simulink model "AIM_v0"  (R2015a)
settings: Solver=ode4  SolverMode=SingleTasking  StartTime=0.0  StopTime=stop_time  FixedStep=1  RelTol=1e-3
undefined symbols (not defined in the file or in its folder): slcm, Target
undefined symbols (not defined in the file): Chaser, Constant
libraries: lib_gravity x6, RotationalDynamics x4, vrlib x3, TranslationalDynamics3DoF x2, Ephemeris_reader x1, Disturbances x1, visualisation x1
settings Model: Creator=bbrito  LastModifiedBy=bbrito
settings DataIOCC: SignalLoggingSaveFormat=ModelDataLogs
settings OptimizationCC: BlockReduction=off  BooleanDataType=off
settings DebuggingCC: SaveWithParameterizedLinksMsg=none  UnderspecifiedInitializationDetection=Classic  MergeDetectMultiDrivingBlocksExec=none  SignalResolutionControl=TryResolveAllWithWarning  MultiTaskDSMMsg=warning  MultiTaskCondExecSysMsg=none
settings HardwareCC: TargetUnknown=on

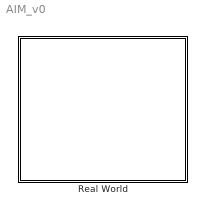
== system AIM_v0 ==
  Real World : Subsystem  TreatAsAtomicUnit=on

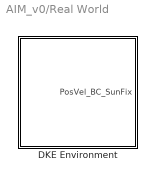
== system AIM_v0/Real World ==
  "DKE Environment " : Subsystem  TreatAsAtomicUnit=on

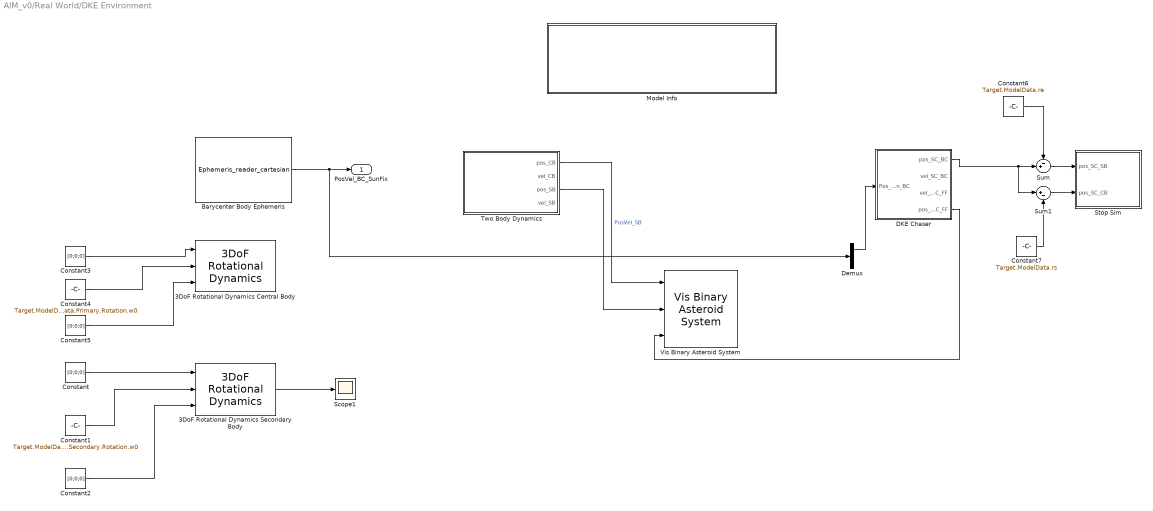
== system AIM_v0/Real World/DKE Environment  ==
  3DoF Rotational Dynamics Central Body : RotationalDynamics/3DoF Rotational Dynamics  I=Target.ModelData.Primary.I
  3DoF Rotational Dynamics Secondary Body : RotationalDynamics/3DoF Rotational Dynamics  I=Target.ModelData.Secondary.I
  Barycenter Body Ephemeris : Ephemeris_reader/Ephemeris_reader_cartesian  traj=Target.ModelData.Primary.Trajectory
  Constant{,2..3,5} (4 alike) : Constant  Value=[0;0;0]
  Constant1 : Constant  Value=Target.ModelData.Secondary.Rotation.w0
  Constant4 : Constant  Value=Target.ModelData.Primary.Rotation.w0
  Constant6 : Constant  Value=Target.ModelData.re
  Constant7 : Constant  Value=Target.ModelData.rs
  DKE Chaser : Subsystem  TreatAsAtomicUnit=on
  Demux : Demux  Outputs=2
  Model Info : Subsystem  LoadFcn=slcm LoadBlock;  InitFcn=slcm('UpdateAllCMBlocksInThisModelInit')  mask(CMBlock){InitialSaveTempField=, InitialBlockCM=, BlockCM=, Frame=on, SaveTempField=, DisplayStringWithTags=|, MaskDisplayString=Copyright ESA, S.A. 2015.\n---------------------------------------------------------------------------\nVersion:0.0          Date:9/11/2015          Author: #BB\nMatlab Ver.: MATLAB 2015a          Project:AIM          Section:TEC-ECN\n---------------------------------------------------------------------------\nAIM target dynamics, HorizontalTextAlignment=Center, LeftAlignmentValue=0.5, SourceBlockDiagram=AIM_v0, TagMaxNumber=20, CMTag1=, CMTag2=, CMTag3=, CMTag4=, CMTag5=, CMTag6=, CMTag7=, CMTag8=, CMTag9=, CMTag10=, CMTag11=, CMTag12=, CMTag13=, CMTag14=, CMTag15=, CMTag16=, CMTag17=, CMTag18=, CMTag19=, CMTag20=}
      mask DisplayStringWithTags=|
      | Copyright ESA, S.A. 2015.
      | ---------------------------------------------------------------------------
      | Version:0.0          Date:9/11/2015          Author: #BB
      | Matlab Ver.: MATLAB 2015a          Project:AIM          Section:TEC-ECN
      | ---------------------------------------------------------------------------
      | AIM target dynamics
      mask prompts: InitialSaveTempField "Simulink:masks:InitialSaveTempField_MP"; InitialBlockCM "Simulink:masks:InitialBlockCM_MP"; BlockCM "Simulink:masks:BlockCM_MP"; Frame "Simulink:masks:Frame_MP"; SaveTempField "Simulink:masks:SaveTempField_MP"; DisplayStringWithTags "Simulink:masks:DisplayStringWithTags_MP"; MaskDisplayString "Simulink:masks:MaskDisplayString_MP"; HorizontalTextAlignment "Simulink:masks:HorizontalTextAlignment_MP"; LeftAlignmentValue "Simulink:masks:LeftAlignmentValue_MP"; SourceBlockDiagram "Simulink:masks:SourceBlockDiagram_MP"; TagMaxNumber "Simulink:masks:TagMaxNumber_MP"; CMTag1 "Simulink:masks:CMTag1_MP"; CMTag2 "Simulink:masks:CMTag2_MP"; CMTag3 "Simulink:masks:CMTag3_MP"; CMTag4 "Simulink:masks:CMTag4_MP"; CMTag5 "Simulink:masks:CMTag5_MP"; CMTag6 "Simulink:masks:CMTag6_MP"; CMTag7 "Simulink:masks:CMTag7_MP"; CMTag8 "Simulink:masks:CMTag8_MP"; CMTag9 "Simulink:masks:CMTag9_MP"; CMTag10 "Simulink:masks:CMTag10_MP"; CMTag11 "Simulink:masks:CMTag11_MP"; CMTag12 "Simulink:masks:CMTag12_MP"; CMTag13 "Simulink:masks:CMTag13_MP"; CMTag14 "Simulink:masks:CMTag14_MP"; CMTag15 "Simulink:masks:CMTag15_MP"; CMTag16 "Simulink:masks:CMTag16_MP"; CMTag17 "Simulink:masks:CMTag17_MP"; CMTag18 "Simulink:masks:CMTag18_MP"; CMTag19 "Simulink:masks:CMTag19_MP"; CMTag20 "Simulink:masks:CMTag20_MP"
      mask help: Simulink:masks:CMBlock_MD
      settings: CopyFcn=slcm CopyBlock;  DeleteFcn=slcm Cancel;  PostSaveFcn=slcm('UpdateAllCMBlocksInThisModel')  NameChangeFcn=slcm Rename;  OpenFcn=slcm
      mask Display: text(str2num(LeftAlignmentValue), 0.5, MaskDisplayString, 'HorizontalAlignment', HorizontalTextAlignment)
  Scope1 : Scope
      settings: YMin=0  YMax=7  SaveName=ScopeData2
  Stop Sim : Subsystem  TreatAsAtomicUnit=on  mask{min_sb=Target.ModelData.Secondary.r0, min_cb=Target.ModelData.Primary.dim}
      mask prompts: min_sb "Minimum Distance SB"; min_cb "Minimum Distance CB"
      mask help:
      | ESA-ESTEC
      | ---------------------------------------------------------------------------
      | Version:0.0          Date:9/11/20015          Author: #BB
      | Matlab version: 2015a          Project: AIM          Division: TEC-ECN
      | ---------------------------------------------------------------------------
      |
      | Stops the simulation if the spacecraft touch the surface of one of the bodys.
      |
      | After this point the gravitational models are not valid anymore.
  Sum : Sum  Inputs=-+|
  Sum1 : Sum  Inputs=|+-
  Two Body Dynamics : Subsystem  TreatAsAtomicUnit=on  mask{g1=Target.ModelData.Primary.GravitationalConstant, g2=Target.ModelData.Secondary.GravitationalConstant}
      mask prompts: g1 "Gravitational Parameter CB"; g2 "Gravitational Parameter SB"
      mask help:
      | ESA-ESTEC
      | ---------------------------------------------------------------------------
      | Version:0.0          Date:9/11/20015          Author: #BB
      | Matlab version: 2015a          Project: AIM          Division: TEC-ECN
      | ---------------------------------------------------------------------------
      |
      | This block implements the Two-Body Problem of the bynary asteroid system.
      |
      | References: Spacecraft Dynamics and Control
      | Author: Marcel J. Sidi
      | Chapter 2.2
  Vis Binary Asteroid System : visualisation/Vis Binary Asteroid System  cb=Target.ModelData.Primary  sb=Target.ModelData.Secondary  cb_w0=Target.ModelData.Primary.Rotation.w0  sb_w0=Target.ModelData.Secondary.Rotation.w0  sc=Chaser.ModelData  cb_dim=Target.ModelData.Primary.dim  sb_dim=Target.ModelData.Secondary.dim  sc_dim=Chaser.ModelData.Parameters.dim
  PosVel_BC_SunFix : Outport
  wires:
  Barycenter Body Ephemeris/1 -> Demux/1, PosVel_BC_SunFix/1
  Constant/1 -> 3DoF Rotational Dynamics Secondary Body/1
  Constant1/1 -> 3DoF Rotational Dynamics Secondary Body/2
  Constant2/1 -> 3DoF Rotational Dynamics Secondary Body/3
  3DoF Rotational Dynamics Secondary Body/1 -> Scope1/1
  Constant3/1 -> 3DoF Rotational Dynamics Central Body/1
  Constant4/1 -> 3DoF Rotational Dynamics Central Body/2
  Constant5/1 -> 3DoF Rotational Dynamics Central Body/3
  Two Body Dynamics/1(pos_CB) -> Vis Binary Asteroid System/1  "PosVel_SB"
  Two Body Dynamics/3(pos_SB) -> Vis Binary Asteroid System/2
  Demux/1 -> DKE Chaser/1(Pos_Sun_BC)
  DKE Chaser/1(pos_SC_BC) -> Sum1/1, Sum/2
  Sum/1 -> Stop Sim/1(pos_SC_SB)
  Constant6/1 -> Sum/1
  Constant7/1 -> Sum1/2
  Sum1/1 -> Stop Sim/2(pos_SC_CB)
  DKE Chaser/4(pos_SC_BC_FF) -> Vis Binary Asteroid System/3

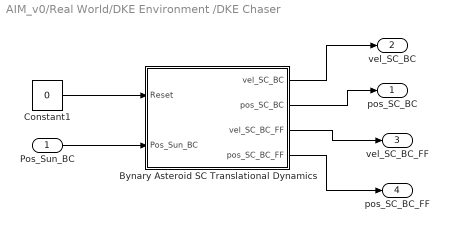
== system AIM_v0/Real World/DKE Environment /DKE Chaser ==
  Pos_Sun_BC : Inport
  Bynary Asteroid SC Translational Dynamics : Subsystem  TreatAsAtomicUnit=on  mask{sphere=Target.ModelData.Primary, rt=Target.ModelData.rt, ellip=Target.ModelData.Secondary, sc=Chaser.ModelData, g=Constant.Gravity, w0=Target.ModelData.Secondary.Rotation.w0}
      mask prompts: sphere "Sphere parameters"; rt "Distance between bodies"; ellip "Ellipsoid parameters"; sc "Spacecraft initial conditions"; g "Gravitational constant"; w0 "Rotational speed"
      mask help:
      | ESA-ESTEC
      | ---------------------------------------------------------------------------
      | Version:0.0          Date:9/11/20015          Author: #BB
      | Matlab version: 2015a          Project: AIM          Division: TEC-ECN
      | ---------------------------------------------------------------------------
      |
      | This block implements the N-Body Problem of the Spacecraft orbiting the bynary asteroid system.
      |
      | The pertubation of the Sun is added as a third bdoy perturbation.
      |
      | The Solar Radiation Pressure is also added.
      |
      | Outputs: pos_SC_BC: Position vector from the barycenter to the spacecraft
      | vel_SC_BC: Velocity vector from the barycenter to the spacecraft
      |
      | References: Orbital Motion in Strongly Perturbed Environments
      | Author: Daniel J. Scheeres
      | Chapter 9.3
  Constant1 : Constant  Value=0
  pos_SC_BC : Outport
  vel_SC_BC : Outport  Port=2
  vel_SC_BC_FF : Outport  Port=3
  pos_SC_BC_FF : Outport  Port=4
  wires:
  Bynary Asteroid SC Translational Dynamics/2(pos_SC_BC) -> pos_SC_BC/1
  Constant1/1 -> Bynary Asteroid SC Translational Dynamics/1(Reset)
  Pos_Sun_BC/1 -> Bynary Asteroid SC Translational Dynamics/2(Pos_Sun_BC)
  Bynary Asteroid SC Translational Dynamics/1(vel_SC_BC) -> vel_SC_BC/1
  Bynary Asteroid SC Translational Dynamics/3(vel_SC_BC_FF) -> vel_SC_BC_FF/1
  Bynary Asteroid SC Translational Dynamics/4(pos_SC_BC_FF) -> pos_SC_BC_FF/1

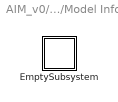
== system AIM_v0/Real World/DKE Environment /Model Info ==
  EmptySubsystem : Subsystem

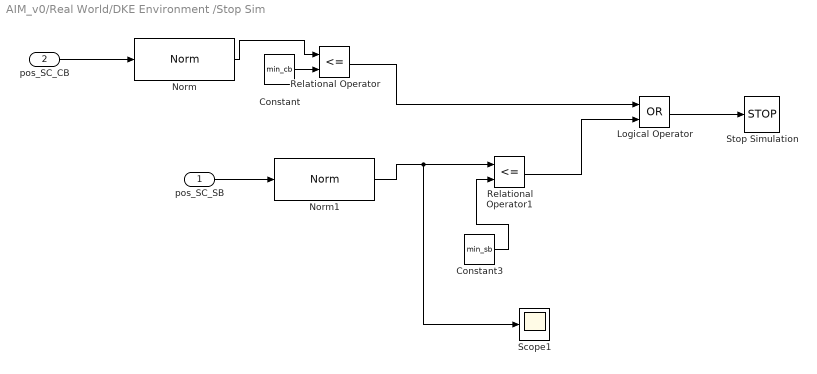
== system AIM_v0/Real World/DKE Environment /Stop Sim ==
  pos_SC_SB : Inport
  pos_SC_CB : Inport  Port=2
  Constant : Constant  Value=min_cb
  Constant3 : Constant  Value=min_sb
  Logical Operator : Logic  Operator=OR  AllPortsSameDT=off  OutDataTypeStr=boolean
  Norm : lib_gravity/Spherical Gravity Acceleration/Norm
  Norm1 : lib_gravity/Spherical Gravity Acceleration/Norm
  Relational Operator : RelationalOperator  Operator=<=  OutDataTypeStr=boolean
  Relational Operator1 : RelationalOperator  Operator=<=  OutDataTypeStr=boolean
  Scope1 : Scope
      settings: YMin=11000  YMax=18000  SaveName=ScopeData4
  Stop Simulation : Stop
  wires:
  Constant/1 -> Relational Operator/2
  Norm/1 -> Relational Operator/1
  Norm1/1 -> Scope1/1, Relational Operator1/1
  Constant3/1 -> Relational Operator1/2
  Relational Operator/1 -> Logical Operator/1
  Relational Operator1/1 -> Logical Operator/2
  pos_SC_SB/1 -> Norm1/1
  pos_SC_CB/1 -> Norm/1
  Logical Operator/1 -> Stop Simulation/1

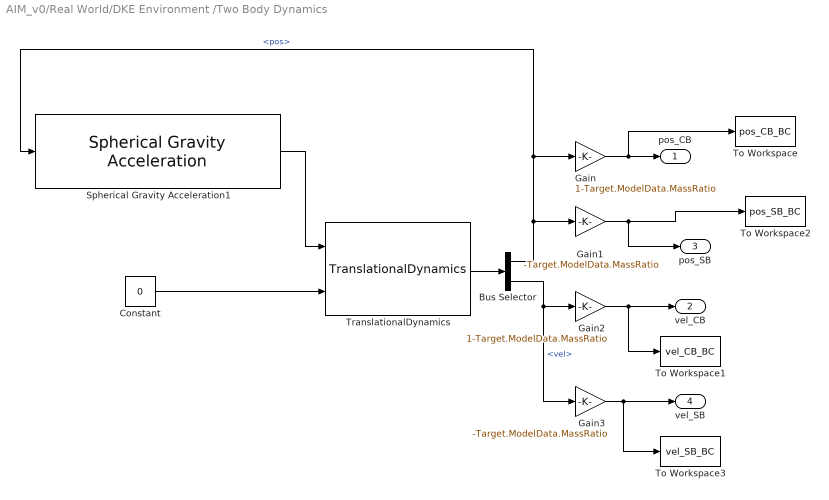
== system AIM_v0/Real World/DKE Environment /Two Body Dynamics ==
  Bus Selector : BusSelector  OutputSignals=pos,vel
  Constant : Constant  Value=0
  Gain : Gain  Gain=1-Target.ModelData.MassRatio
  Gain1 : Gain  Gain=-Target.ModelData.MassRatio
  Gain2 : Gain  Gain=1-Target.ModelData.MassRatio
  Gain3 : Gain  Gain=-Target.ModelData.MassRatio
  Spherical Gravity Acceleration1 : lib_gravity/Spherical Gravity Acceleration  u=g1+g2
  To Workspace : ToWorkspace  VariableName=pos_CB_BC  SaveFormat=Timeseries  SampleTime=-1
  To Workspace1 : ToWorkspace  VariableName=vel_CB_BC  SaveFormat=Timeseries  SampleTime=-1
  To Workspace2 : ToWorkspace  VariableName=pos_SB_BC  SaveFormat=Timeseries  SampleTime=-1
  To Workspace3 : ToWorkspace  VariableName=vel_SB_BC  SaveFormat=Timeseries  SampleTime=-1
  TranslationalDynamics : TranslationalDynamics3DoF/TranslationalDynamics  v0=Target.ModelData.v0  x0=Target.ModelData.x0
  pos_CB : Outport
  vel_CB : Outport  Port=2
  pos_SB : Outport  Port=3
  vel_SB : Outport  Port=4
  wires:
  Constant/1 -> TranslationalDynamics/2
  TranslationalDynamics/1 -> Bus Selector/1
  Bus Selector/1 -> Gain1/1, Gain/1, Spherical Gravity Acceleration1/1  "<pos>"
  Spherical Gravity Acceleration1/1 -> TranslationalDynamics/1
  Gain/1 -> To Workspace/1, pos_CB/1
  Gain1/1 -> pos_SB/1, To Workspace2/1
  Gain2/1 -> To Workspace1/1, vel_CB/1
  Bus Selector/2 -> Gain3/1, Gain2/1  "<vel>"
  Gain3/1 -> To Workspace3/1, vel_SB/1

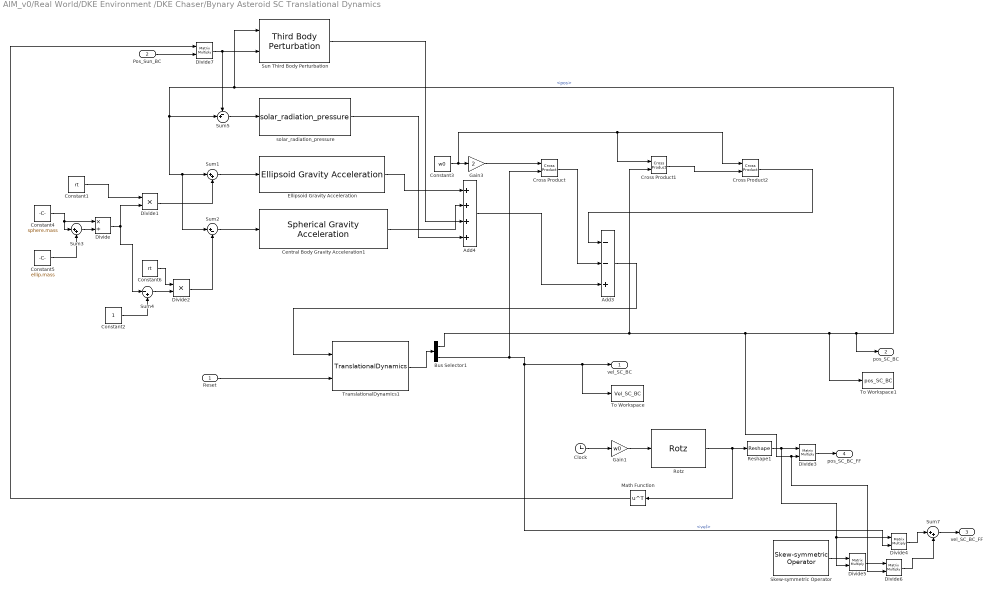
== system AIM_v0/Real World/DKE Environment /DKE Chaser/Bynary Asteroid SC Translational Dynamics ==
  Reset : Inport
  Pos_Sun_BC : Inport  Port=2
  Add3 : Sum  Inputs=--+
  Add4 : Sum  Inputs=++++
  Bus Selector1 : BusSelector  OutputSignals=pos,vel
  Central Body Gravity Acceleration1 : lib_gravity/Spherical Gravity Acceleration  u=sphere.mass*g
  Clock : Clock
  Constant1 : Constant  Value=rt
  Constant2 : Constant
  Constant3 : Constant  Value=w0
  Constant4 : Constant  Value=sphere.mass
  Constant5 : Constant  Value=ellip.mass
  Constant6 : Constant  Value=rt
  Cross Product : vrlib/Utilities/Cross Product
  Cross Product1 : vrlib/Utilities/Cross Product
  Cross Product2 : vrlib/Utilities/Cross Product
  Divide : Product  Inputs=*/
  Divide1 : Product  Inputs=**
  Divide2 : Product  Inputs=**
  Divide{3..7} (5 alike) : Product  Inputs=**  Multiplication=Matrix(*)
  Ellipsoid Gravity Acceleration : lib_gravity/Ellipsoid Gravity Acceleration  dim=ellip.dim  r0=ellip.r0  u=ellip.mass*g
  Gain1 : Gain  Gain=w0
  Gain3 : Gain  Gain=2
  Math Function : Math  Operator=transpose  SaturateOnIntegerOverflow=on
  Reshape1 : Reshape  OutputDimensionality=Customize  OutputDimensions=[3,3]
  Rotz : RotationalDynamics/Rotz
  Skew-symmetric Operator : RotationalDynamics/Skew-symmetric Operator  omega=Target.ModelData.Secondary.Rotation.w0
  Sum1 : Sum  Inputs=|++
  Sum2 : Sum  Inputs=|+-
  Sum3 : Sum  Inputs=|++
  Sum4 : Sum  Inputs=|-+
  Sum5 : Sum  Inputs=-+|
  Sum7 : Sum  Inputs=|++
  Sun Third Body Perturbation : lib_gravity/Third Body Perturbation  u=Constant.SunGravity
  To Workspace : ToWorkspace  VariableName=Vel_SC_BC  SaveFormat=Timeseries  SampleTime=-1
  To Workspace1 : ToWorkspace  VariableName=pos_SC_BC  SaveFormat=Timeseries  SampleTime=-1
  TranslationalDynamics1 : TranslationalDynamics3DoF/TranslationalDynamics  v0=sc.v0_BC  x0=sc.x0_BC
  solar_radiation_pressure : Disturbances/solar_radiation_pressure  solar_const=Chaser.ModelData.Parameters.solar_const  astr_unit=Chaser.ModelData.Parameters.astr_unit  cross_area=Chaser.ModelData.Parameters.area  solar_rad_press_coef=Chaser.ModelData.Parameters.rad_press_coef  light_speed=Chaser.ModelData.Parameters.light_speed  sc_mass=Chaser.ModelData.Parameters.mass  timestep=Sim.Ts
  vel_SC_BC : Outport
  pos_SC_BC : Outport  Port=2
  vel_SC_BC_FF : Outport  Port=3
  pos_SC_BC_FF : Outport  Port=4
  wires:
  Gain1/1 -> Rotz/1
  Clock/1 -> Gain1/1
  Divide6/1 -> Sum7/2
  Divide4/1 -> Sum7/1
  Divide5/1 -> Divide6/1
  Skew-symmetric Operator/1 -> Divide5/1
  Reshape1/1 -> Divide3/1, Divide5/2, Divide4/1
  Rotz/1 -> Math Function/1, Reshape1/1
  Reset/1 -> TranslationalDynamics1/2
  Divide2/1 -> Sum2/2
  Constant6/1 -> Divide2/1
  Sum4/1 -> Divide2/2
  Constant2/1 -> Sum4/2
  Constant1/1 -> Divide1/1
  Divide/1 -> Divide1/2, Sum4/1
  Divide1/1 -> Sum1/2
  Sum3/1 -> Divide/2
  Constant5/1 -> Sum3/2
  Constant4/1 -> Sum3/1, Divide/1
  Add3/1 -> TranslationalDynamics1/1
  Bus Selector1/1 -> Divide3/2, Divide6/2, To Workspace1/1, pos_SC_BC/1, Sun Third Body Perturbation/1, Sum5/2, Sum1/1, Sum2/1, Cross Product1/2  "<pos>"
  Bus Selector1/2 -> Cross Product/2, To Workspace/1, vel_SC_BC/1, Divide4/2  "<vel>"
  TranslationalDynamics1/1 -> Bus Selector1/1
  Ellipsoid Gravity Acceleration/1 -> Add4/1
  Sum2/1 -> Central Body Gravity Acceleration1/1
  Add4/1 -> Add3/3
  Central Body Gravity Acceleration1/1 -> Add4/2
  Sum1/1 -> Ellipsoid Gravity Acceleration/1
  Cross Product/1 -> Add3/2
  Cross Product2/1 -> Add3/1
  Cross Product1/1 -> Cross Product2/2
  Constant3/1 -> Gain3/1, Cross Product2/1, Cross Product1/1
  Gain3/1 -> Cross Product/1
  Pos_Sun_BC/1 -> Divide7/2
  Math Function/1 -> Divide7/1
  Divide7/1 -> Sum5/1, Sun Third Body Perturbation/2
  Sum5/1 -> solar_radiation_pressure/1
  Sum7/1 -> vel_SC_BC_FF/1
  Divide3/1 -> pos_SC_BC_FF/1
  solar_radiation_pressure/1 -> Add4/4
  Sun Third Body Perturbation/1 -> Add4/3

== system AIM_v0/Real World/DKE Environment /Model Info/EmptySubsystem ==
